simulink model "hw2_eserc_5_simulink"  (R2023b)
settings: Solver=FixedStepAuto  StartTime=0.0  StopTime=20  FixedStep=1/fs  RelTol=1e-3
undefined symbols (not defined in the file or in its folder): fs, k1, k2, k3, qi
libraries: robotmobilelib x1
settings Model: Creator=lalla  LastModifiedBy=lalla

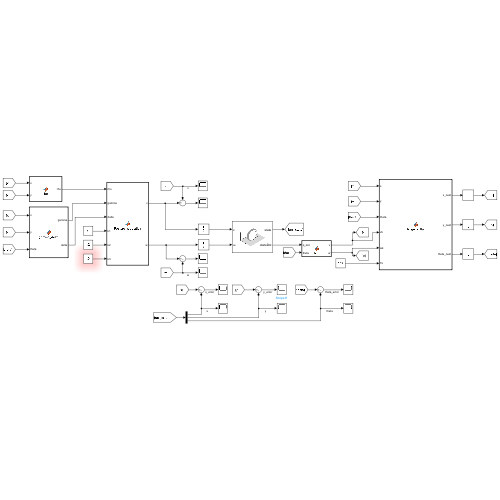
[thumbnail: Simulink's stored preview of the top-level diagram]
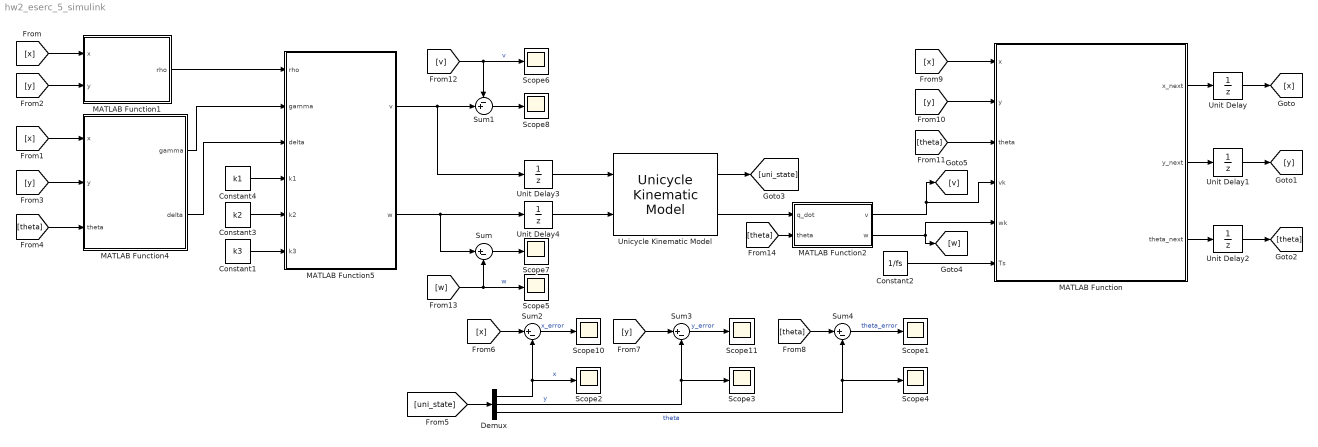
== system hw2_eserc_5_simulink ==
  Constant1 : Constant  Value=k3
  Constant2 : Constant  Value=1/fs
  Constant3 : Constant  Value=k2
  Constant4 : Constant  Value=k1
  Demux : Demux  Outputs=3
  MATLAB Function : MATLAB Function  Tag=inte  TreatAsAtomicUnit=on
  MATLAB Function1 : MATLAB Function  TreatAsAtomicUnit=on
  MATLAB Function2 : MATLAB Function  TreatAsAtomicUnit=on
  MATLAB Function4 : MATLAB Function  TreatAsAtomicUnit=on
  MATLAB Function5 : MATLAB Function  TreatAsAtomicUnit=on
  Scope{1..8,10..11} (10 alike) : Scope
  Sum{,2..4} (4 alike) : Sum  Inputs=|+-
  Sum1 : Sum  Inputs=-+|
  Unicycle Kinematic Model : robotmobilelib/Unicycle Kinematic Model  VehicleInputs=Vehicle Speed & Heading Angular Velocity  WheelRadius=0.1  WheelSpeedRange=[-Inf Inf]  InitialState=qi  SimulateUsing=Interpreted execution
  Unit Delay : UnitDelay  InitialCondition=qi(1)  SampleTime=-1  HasFrameUpgradeWarning=on
  Unit Delay1 : UnitDelay  InitialCondition=qi(2)  SampleTime=-1  HasFrameUpgradeWarning=on
  Unit Delay2 : UnitDelay  InitialCondition=qi(3)  SampleTime=-1  HasFrameUpgradeWarning=on
  Unit Delay3 : UnitDelay  SampleTime=-1  HasFrameUpgradeWarning=on
  Unit Delay4 : UnitDelay  SampleTime=-1  HasFrameUpgradeWarning=on
  wires:
  MATLAB Function/1(x_next) -> Unit Delay/1
  MATLAB Function/2(y_next) -> Unit Delay1/1
  MATLAB Function4/1(gamma) -> MATLAB Function5/2(gamma)
  MATLAB Function1/1(rho) -> MATLAB Function5/1(rho)
  MATLAB Function4/2(delta) -> MATLAB Function5/3(delta)
  Constant1/1 -> MATLAB Function5/6(k3)
  MATLAB Function5/1(v) -> Unit Delay3/1, Sum1/2
  Constant2/1 -> MATLAB Function/6(Ts)
  [x] -> MATLAB Function1/1(x)
  [x] -> MATLAB Function4/1(x)
  [y] -> MATLAB Function1/2(y)
  [y] -> MATLAB Function4/2(y)
  [theta] -> MATLAB Function4/3(theta)
  Constant3/1 -> MATLAB Function5/5(k2)
  Constant4/1 -> MATLAB Function5/4(k1)
  Unit Delay3/1 -> Unicycle Kinematic Model/1
  Unit Delay4/1 -> Unicycle Kinematic Model/2
  Sum/1 -> Scope7/1
  Sum1/1 -> Scope8/1
  MATLAB Function5/2(w) -> Unit Delay4/1, Sum/1
  Demux/1 -> Sum2/2, Scope2/1  "x"
  Demux/2 -> Scope3/1, Sum3/2  "y"
  Sum2/1 -> Scope10/1  "x_error"
  Sum3/1 -> Scope11/1  "y_error"
  Demux/3 -> Sum4/2, Scope4/1  "theta"
  Sum4/1 -> Scope1/1  "theta_error"
  MATLAB Function/3(theta_next) -> Unit Delay2/1
  Unicycle Kinematic Model/1 -> [uni_state]
  [uni_state] -> Demux/1
  [x] -> Sum2/1
  [y] -> Sum3/1
  [theta] -> Sum4/1
  Unit Delay/1 -> [x]
  Unit Delay1/1 -> [y]
  Unit Delay2/1 -> [theta]
  [x] -> MATLAB Function/1(x)
  [y] -> MATLAB Function/2(y)
  [theta] -> MATLAB Function/3(theta)
  [v] -> Scope6/1, Sum1/1  "v"
  [w] -> Scope5/1, Sum/2  "w"
  MATLAB Function2/2(w) -> MATLAB Function/5(wk), [w]
  Unicycle Kinematic Model/2 -> MATLAB Function2/1(q_dot)
  MATLAB Function2/1(v) -> [v], MATLAB Function/4(vk)
  [theta] -> MATLAB Function2/2(theta)

== matlab function hw2_eserc_5_simulink/MATLAB Function1 ==
  data: x input; rho output; y input
function rho = rho(x,y)
rho = sqrt(x^2 + y^2);

== matlab function hw2_eserc_5_simulink/MATLAB Function ==
  data: x input; x_next output; y input; theta input; vk input; wk input; Ts input; y_next output; theta_next output
function [x_next,y_next,theta_next] = Ruge_kutta(x,y,theta,vk,wk,Ts)
x_next = x +vk*Ts*cos(theta+wk*Ts/2);
y_next = y +vk*Ts*sin(theta+wk*Ts/2);
theta_next = theta + wk*Ts;

== matlab function hw2_eserc_5_simulink/MATLAB Function2 ==
  data: q_dot input; v output; w output; theta input
function [v,w] = fcn(q_dot,theta)
v= q_dot(1)/cos(theta);
w= q_dot(3);

== matlab function hw2_eserc_5_simulink/MATLAB Function4 ==
  data: x input; gamma output; y input; theta input; delta output
function [gamma,delta] = gamma_delta(x,y,theta)
gamma = atan2(y,x) - theta + pi;
delta = atan2(y,x) + pi;

== matlab function hw2_eserc_5_simulink/MATLAB Function5 ==
  data: rho input; v output; gamma input; delta input; k1 input; k2 input; k3 input; w output
function [v,w] = Posture_regulation(rho,gamma,delta,k1,k2,k3)
v=k1*rho*cos(gamma);
w=k2*gamma+k1*sin(gamma)*cos(gamma)*(1+k3*delta/gamma);
